simulink model "DT"  (R2025b)
settings: Solver=ode5  StartTime=0.0  StopTime=inf  RelTol=1e-3
InitFcn:
  | PLC_IP = "10.10.6.1";
  | port_num = 502;
  | 
  | 
  | load("macierze_do_modelu.mat")
undefined symbols (not defined in the file or in its folder): dol_p1, dol_p2, dol_p3, flows_diff, gora_p1, gora_p2, gora_p3, lvls, M_cofka, M_pump_A1, online, pompa_sterowanie, pump_a1_delay_a, pump_a1_delay_b, pump_a2_delay_a, pump_a2_delay_b, R1_K_dol, R1_K_gora, R1_sterowanie, R2_K_dol, R2_K_gora, R2_od_dolu, R2_od_gory, R2_sterowanie, R3, R4, R5, R6, R7, rozgalezienie_h1_dol, rozgalezienie_h1_gora, rozgalezienie_h2_dol, rozgalezienie_h2_gora, rozgalezienie_korekta_A1_dol, rozgalezienie_korekta_A2_dol, sterowanie, V_max, V_out_max
libraries: modbuslib x5, simulink x2, sldrtlib x1
settings Model: ParamWorkspaceSource=ReferencedWorkspace  TunableVars=R4,R3,R5,R6,R7,R8,R1_sterowanie,R2_sterowanie,pompa_sterowanie  TunableVarsStorageClass=Auto,Auto,Auto,Auto,Auto,Auto,Auto,Auto,Auto  TunableVarsTypeQualifier=,,,,,,,,  Creator=Ania  LastModifiedBy=student
settings DebuggingCC: UnderspecifiedInitializationDetection=Classic  MergeDetectMultiDrivingBlocksExec=none
settings HardwareCC: ProdBitPerLong=64.0  ProdHWDeviceType=Intel->x86-64 (Linux 64)
settings ModelReferenceCC: PropagateSignalLabelsOutOfModel=off
settings RTWCC: SystemTargetFile=sldrt.tlc  TemplateMakefile=sldrt.tmf  RTWCompilerOptimization=on  Description=Simulink Desktop Real-Time
settings CodeAppCC: MaxIdLength=95.0
settings SimulinkDesktopRealTimeCC: ExtModeTransport=0.0  ExtModeStaticAllocSize=1000000.0  TargetLibSuffix=_sldrt.a  TargetPreCompLibLocation=C:\Program Files\MATLAB\R2025b\toolbox\sldrt\lib\win64  MultiwordLength=2048.0  DynamicStringBufferSize=256.0  ParMdlRefBuildCompliant=on  PreserveMATLABNamespacesInGeneratedCode=on  SubcomponentCodeInterfacePackaging=Reusable function

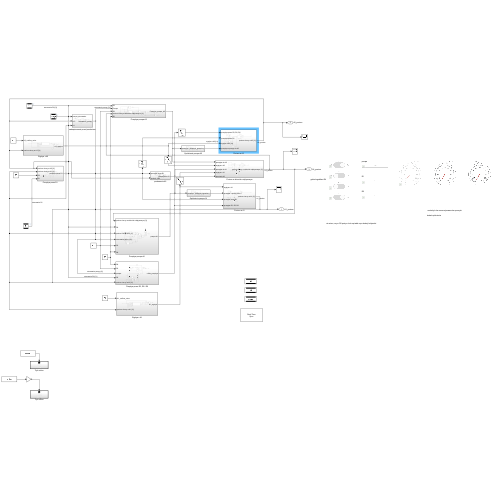
[thumbnail: Simulink's stored preview of the top-level diagram]
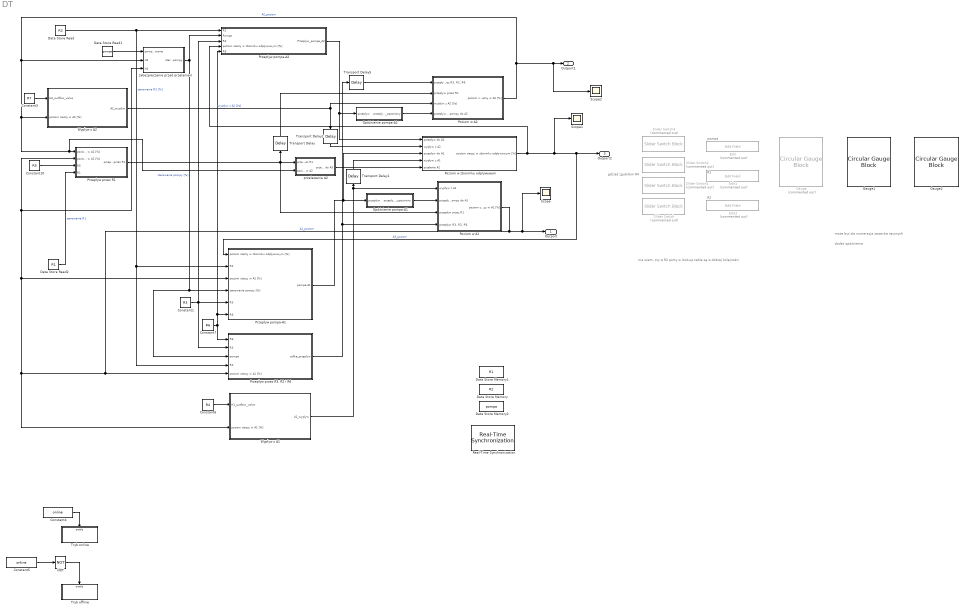
== system DT ==
  note: nie wiem, czy w R2 porty w look-up table są w dobrej kolejności
  note: dodać opóźnienia
  note: gdzieś zgubiłam R4
  note: R2
  note: R1
  note: pompa
  note: może być zła numeracja zaworów ręcznych
  Constant1 : Constant  Value=R3  OutDataTypeStr=boolean
  Constant10 : Constant  Value=R5  OutDataTypeStr=boolean
  Constant3 : Constant  Value=R7  OutDataTypeStr=boolean
  Constant4 : Constant  Value=online  OutDataTypeStr=boolean
  Constant5 : Constant  Value=online  OutDataTypeStr=boolean
  Constant6 : Constant  Value=R4  OutDataTypeStr=boolean
  Constant7 : Constant  Value=R6  OutDataTypeStr=boolean
  Data Store Memory : DataStoreMemory  DataStoreName=R2  WriteAfterWriteMsg=warning  ShowAdditionalParam=off
  Data Store Memory1 : DataStoreMemory  DataStoreName=R1  WriteAfterWriteMsg=warning  ShowAdditionalParam=off
  Data Store Memory2 : DataStoreMemory  DataStoreName=pompa  WriteAfterWriteMsg=warning  ShowAdditionalParam=off
  Data Store Read : DataStoreRead  DataStoreName=R2  IndexOptions=Index vector (dialog)  Indices=1  OutputSizes=1
  Data Store Read1 : DataStoreRead  DataStoreName=pompa  IndexOptions=Index vector (dialog)  Indices=1  OutputSizes=1
  Data Store Read2 : DataStoreRead  DataStoreName=R1  IndexOptions=Index vector (dialog)  Indices=1  OutputSizes=1
  Edit : EditField  Commented=on  LabelPosition=Hide  ShowInitialText=on  Alignment=Center
  Edit1 : EditField  Commented=on  LabelPosition=Hide  ShowInitialText=on  Alignment=Center
  Edit2 : EditField  Commented=on  LabelPosition=Hide  ShowInitialText=on  Alignment=Center
  Gauge : CircularGaugeBlock  Commented=on  FontColor=[0.0, 0.0, 0.0]
  Gauge1 : CircularGaugeBlock  FontColor=[0.0, 0.0, 0.0]
  Gauge2 : CircularGaugeBlock  FontColor=[0.0, 0.0, 0.0]
  NOT : Logic  Operator=NOT  IconShape=distinctive  AllPortsSameDT=off  OutDataTypeStr=boolean
  Opóźnienie pompa-A1 : Subsystem
  Opóźnienie pompa-A2 : Subsystem
  Poziom w A1 : Subsystem
  Poziom w A2 : Subsystem
  Poziom w zbiorniku odplywowym : Subsystem
  Przepływ pompa-A1 : Subsystem
  Przepływ pompa-A2 : Subsystem
  Przepływ przez R1 : Subsystem
  "Przepływ przez R3, R2 i R6" : Subsystem
  Real-Time Synchronization : sldrtlib/Real-Time Synchronization  SampleTime=0.1  MaxMissedTicks=5000  ShowMissedTicks=off  YieldWhenWaiting=off
  Scope : Scope
      settings: DataLoggingSaveFormat=Array
  Scope1 : Scope
      settings: DataLoggingSaveFormat=Array
  Scope2 : Scope
      settings: DataLoggingVariableName=ScopeData2  DataLoggingSaveFormat=Array
  Slider Switch{,1..2,4} (4 alike) : SliderSwitchBlock  Commented=on
  Transport Delay : TransportDelay  DelayTime=1.65
  Transport Delay1 : TransportDelay  DelayTime=1.15
  Transport Delay2 : TransportDelay  DelayTime=0.9
  Transport Delay5 : TransportDelay  DelayTime=2
  Tryb offline : Subsystem  TreatAsAtomicUnit=on
  Tryb online : Subsystem  TreatAsAtomicUnit=on
  Wypływ z A1 : Subsystem
  Wypływ z A2 : Subsystem
  przelewanie A2 : Subsystem
  zabezpieczenie przed przelaniem : Subsystem
  Outport : Outport  SignalName=A1_poziom
  Outport1 : Outport  Port=2  SignalName=A2_poziom
  Outport2 : Outport  Port=3  SignalName=A3_poziom
  wires:
  Data Store Read/1 -> "Przepływ przez R3, R2 i R6"/4(R2), Przepływ pompa-A1/2(R2), Przepływ pompa-A2/1(R2)  "sterowanie R2 [%]"
  Przepływ pompa-A2/1(Przeplyw_pompa_A2) -> Poziom w zbiorniku odplywowym/1(przepływ do A2), Opóźnienie pompa-A2/1(przeplyw)
  Wypływ z A2/1(A2_wypływ) -> Poziom w A2/3(wypływ z A2 [l/s]), Transport Delay2/1  "wypływ z A2 [l/s]"
  Constant3/1 -> Wypływ z A2/1(H2_outflow_valve)
  Wypływ z A1/1(A1_wyplyw) -> Poziom w A1/1(wypływ z A1), Transport Delay1/1
  Constant6/1 -> Wypływ z A1/1(H1_outflow_valve)
  "Przepływ przez R3, R2 i R6"/1(cofka_przeplyw) -> Transport Delay5/1, Poziom w A1/4("przepływ R3, R2, R6")
  Constant7/1 -> "Przepływ przez R3, R2 i R6"/1(R6), Przepływ pompa-A2/5(R6), Przepływ pompa-A1/6(R6)
  Przepływ pompa-A1/1(pompa-A1) -> Poziom w zbiorniku odplywowym/3(przepływ do A1), Opóźnienie pompa-A1/1(przeplyw)
  Data Store Read2/1 -> Przepływ przez R1/4(R1)  "sterowanie R1"
  Przepływ przez R1/1(przepływ przez R1) -> Transport Delay/1, Poziom w A1/3(przepływ przez R1), przelewanie A2/1(przepływ przez R1)
  Constant10/1 -> Przepływ przez R1/3(R5)
  Poziom w A1/1(poziom cieczy w A1 [%]) -> "Przepływ przez R3, R2 i R6"/5(poziom cieczy w A1 [%]), Przepływ przez R1/2(poziom cieczy w A1 [%]), zabezpieczenie przed przelaniem/3(H1), Przepływ pompa-A1/3(poziom cieczy w A1 [%]), Wypływ z A1/2(poziom cieczy w A1 [%]), Scope/1, Outport/1  "A1_poziom"
  Poziom w A2/1(poziom cieczy w A2 [%]) -> Scope2/1, Outport1/1, Wypływ z A2/2(poziom cieczy w A2 [%]), Przepływ przez R1/1(poziom cieczy w A2 [%]), przelewanie A2/2(poziom w A2), zabezpieczenie przed przelaniem/2(H2)  "A2_poziom"
  Poziom w zbiorniku odplywowym/1(poziom cieczy w zbiorniku odpływowym [%]) -> Scope1/1, Przepływ pompa-A1/1(poziom cieczy w zbiorniku odpływowym [%]), Outport2/1, Przepływ pompa-A2/4(poziom cieczy w zbiorniku odpływowym [%])  "A3_poziom"
  Constant1/1 -> "Przepływ przez R3, R2 i R6"/2(R3), Przepływ pompa-A2/3(R3), Przepływ pompa-A1/5(R3)
  zabezpieczenie przed przelaniem/1(sterowanie_pompy) -> "Przepływ przez R3, R2 i R6"/3(pompa), Przepływ pompa-A1/4(sterowanie pompy [%]), Przepływ pompa-A2/2(Pompa)  "sterowanie pompy [%]"
  Data Store Read1/1 -> zabezpieczenie przed przelaniem/1(pompa_sterowanie)
  przelewanie A2/1(przepływ do A3) -> Poziom w zbiorniku odplywowym/5(przelanie A2)
  Transport Delay/1 -> Poziom w A2/2(przepływ przez R1)
  Transport Delay1/1 -> Poziom w zbiorniku odplywowym/4(wypływ z A1)
  Transport Delay2/1 -> Poziom w zbiorniku odplywowym/2(wypływ z A2)
  Opóźnienie pompa-A2/1(przeplyw_opozniony) -> Poziom w A2/4(przepływ z pompy do A2)
  Opóźnienie pompa-A1/1(przeplyw_opozniony) -> Poziom w A1/2(przepływ z pompy do A1)
  Transport Delay5/1 -> Poziom w A2/1("przepływ przez R3, R2, R6")
  Constant4/1 -> Tryb online/Enable
  NOT/1 -> Tryb offline/Enable
  Constant5/1 -> NOT/1

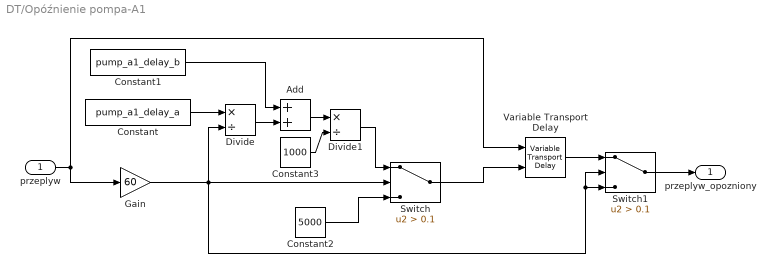
== system DT/Opóźnienie pompa-A1 ==
  przeplyw : Inport
  Add : Sum
  Constant : Constant  Value=pump_a1_delay_a
  Constant1 : Constant  Value=pump_a1_delay_b
  Constant2 : Constant  Value=5000
  Constant3 : Constant  Value=1000
  Divide : Product  Inputs=*/
  Divide1 : Product  Inputs=*/
  Gain : Gain  Gain=60
  Switch : Switch  Criteria=u2 > Threshold  Threshold=0.1  SaturateOnIntegerOverflow=off  InputSameDT=off
  Switch1 : Switch  Criteria=u2 > Threshold  Threshold=0.1  SaturateOnIntegerOverflow=off  InputSameDT=off
  Variable Transport Delay : VariableTransportDelay  VariableDelayType=Variable transport delay  MaximumDelay=5000
  przeplyw_opozniony : Outport
  wires:
  Constant/1 -> Divide/1
  przeplyw/1 -> Gain/1, Variable Transport Delay/1
  Divide/1 -> Add/2
  Constant1/1 -> Add/1
  Constant2/1 -> Switch/3
  Switch/1 -> Variable Transport Delay/2
  Add/1 -> Divide1/1
  Divide1/1 -> Switch/1
  Constant3/1 -> Divide1/2
  Gain/1 -> Switch/2, Switch1/3, Switch1/2, Divide/2
  Variable Transport Delay/1 -> Switch1/1
  Switch1/1 -> przeplyw_opozniony/1

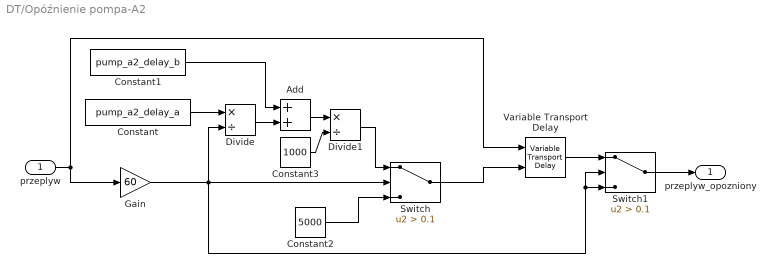
== system DT/Opóźnienie pompa-A2 ==
  przeplyw : Inport
  Add : Sum
  Constant : Constant  Value=pump_a2_delay_a
  Constant1 : Constant  Value=pump_a2_delay_b
  Constant2 : Constant  Value=5000
  Constant3 : Constant  Value=1000
  Divide : Product  Inputs=*/
  Divide1 : Product  Inputs=*/
  Gain : Gain  Gain=60
  Switch : Switch  Criteria=u2 > Threshold  Threshold=0.1  SaturateOnIntegerOverflow=off  InputSameDT=off
  Switch1 : Switch  Criteria=u2 > Threshold  Threshold=0.1  SaturateOnIntegerOverflow=off  InputSameDT=off
  Variable Transport Delay : VariableTransportDelay  VariableDelayType=Variable transport delay  MaximumDelay=5000
  przeplyw_opozniony : Outport
  wires:
  Switch1/1 -> przeplyw_opozniony/1
  Variable Transport Delay/1 -> Switch1/1
  Gain/1 -> Divide/2, Switch1/2, Switch1/3, Switch/2
  Constant3/1 -> Divide1/2
  Divide1/1 -> Switch/1
  Add/1 -> Divide1/1
  Switch/1 -> Variable Transport Delay/2
  Constant2/1 -> Switch/3
  Constant1/1 -> Add/1
  Divide/1 -> Add/2
  przeplyw/1 -> Variable Transport Delay/1, Gain/1
  Constant/1 -> Divide/1

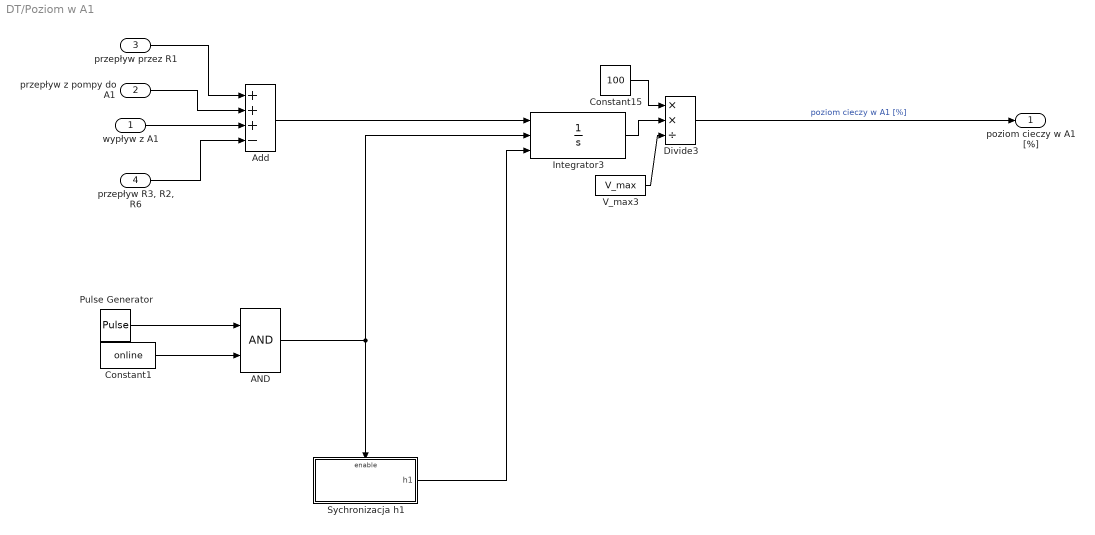
== system DT/Poziom w A1 ==
  wypływ z A1 : Inport
  przepływ z pompy do A1 : Inport  Port=2
  przepływ przez R1 : Inport  Port=3
  "przepływ R3, R2, R6" : Inport  Port=4
  AND : Logic  IconShape=distinctive  AllPortsSameDT=off  OutDataTypeStr=boolean
  Add : Sum  Inputs=+++-
  Constant1 : Constant  Value=online  OutDataTypeStr=boolean
  Constant15 : Constant  Value=100
  Divide3 : Product  Inputs=**/
  Integrator3 : Integrator  ExternalReset=rising  InitialConditionSource=external  LimitOutput=on  UpperSaturationLimit=V_max  LowerSaturationLimit=0
  Pulse Generator : DiscretePulseGenerator  PulseType=Time based  Period=60  PulseWidth=5
  Sychronizacja h1 : Subsystem  TreatAsAtomicUnit=on
  V_max3 : Constant  Value=V_max
  poziom cieczy w A1 [%] : Outport
  wires:
  wypływ z A1/1 -> Add/3
  przepływ z pompy do A1/1 -> Add/2
  Add/1 -> Integrator3/1
  Integrator3/1 -> Divide3/2
  Constant15/1 -> Divide3/1
  Divide3/1 -> poziom cieczy w A1 [%]/1  "poziom cieczy w A1 [%]"
  V_max3/1 -> Divide3/3
  "przepływ R3, R2, R6"/1 -> Add/4
  przepływ przez R1/1 -> Add/1
  Sychronizacja h1/1(h1) -> Integrator3/3
  Constant1/1 -> AND/2
  AND/1 -> Integrator3/2, Sychronizacja h1/Enable
  Pulse Generator/1 -> AND/1

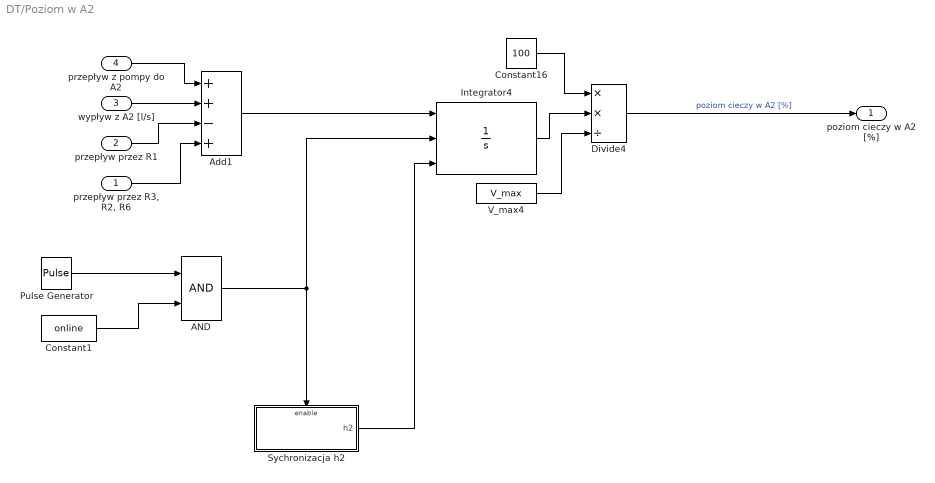
== system DT/Poziom w A2 ==
  "przepływ przez R3, R2, R6" : Inport
  przepływ przez R1 : Inport  Port=2
  wypływ z A2 [l/s] : Inport  Port=3
  przepływ z pompy do A2 : Inport  Port=4
  AND : Logic  IconShape=distinctive  AllPortsSameDT=off  OutDataTypeStr=boolean
  Add1 : Sum  Inputs=++-+
  Constant1 : Constant  Value=online  OutDataTypeStr=boolean
  Constant16 : Constant  Value=100
  Divide4 : Product  Inputs=**/
  Integrator4 : Integrator  ExternalReset=rising  InitialConditionSource=external  LimitOutput=on  UpperSaturationLimit=V_max  LowerSaturationLimit=0
  Pulse Generator : DiscretePulseGenerator  PulseType=Time based  Period=60  PulseWidth=5
  Sychronizacja h2 : Subsystem  TreatAsAtomicUnit=on
  V_max4 : Constant  Value=V_max
  poziom cieczy w A2 [%] : Outport
  wires:
  "przepływ przez R3, R2, R6"/1 -> Add1/4
  V_max4/1 -> Divide4/3
  Integrator4/1 -> Divide4/2
  wypływ z A2 [l/s]/1 -> Add1/2
  Divide4/1 -> poziom cieczy w A2 [%]/1  "poziom cieczy w A2 [%]"
  Add1/1 -> Integrator4/1
  Constant16/1 -> Divide4/1
  przepływ z pompy do A2/1 -> Add1/1
  przepływ przez R1/1 -> Add1/3
  Pulse Generator/1 -> AND/1
  Constant1/1 -> AND/2
  AND/1 -> Integrator4/2, Sychronizacja h2/Enable
  Sychronizacja h2/1(h2) -> Integrator4/3

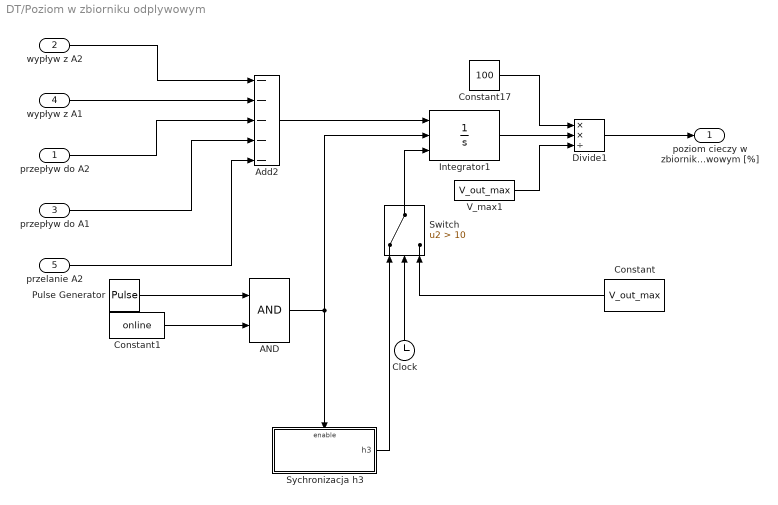
== system DT/Poziom w zbiorniku odplywowym ==
  przepływ do A2 : Inport
  wypływ z A2 : Inport  Port=2
  przepływ do A1 : Inport  Port=3
  wypływ z A1 : Inport  Port=4
  przelanie A2 : Inport  Port=5
  AND : Logic  IconShape=distinctive  AllPortsSameDT=off  OutDataTypeStr=boolean
  Add2 : Sum  Inputs=-----
  Clock : Clock
  Constant : Constant  Value=V_out_max
  Constant1 : Constant  Value=online  OutDataTypeStr=boolean
  Constant17 : Constant  Value=100
  Divide1 : Product  Inputs=**/
  Integrator1 : Integrator  ExternalReset=rising  InitialConditionSource=external  InitialCondition=V_out_max  LimitOutput=on  UpperSaturationLimit=V_out_max  LowerSaturationLimit=0
  Pulse Generator : DiscretePulseGenerator  PulseType=Time based  Period=60  PulseWidth=5
  Switch : Switch  Criteria=u2 > Threshold  Threshold=10  SaturateOnIntegerOverflow=off  InputSameDT=off
  Sychronizacja h3 : Subsystem  TreatAsAtomicUnit=on
  V_max1 : Constant  Value=V_out_max  OutDataTypeStr=double
  poziom cieczy w zbiorniku odpływowym [%] : Outport
  wires:
  Add2/1 -> Integrator1/1
  V_max1/1 -> Divide1/3
  Integrator1/1 -> Divide1/2
  przepływ do A1/1 -> Add2/4
  Constant17/1 -> Divide1/1
  wypływ z A1/1 -> Add2/2
  Divide1/1 -> poziom cieczy w zbiorniku odpływowym [%]/1
  przepływ do A2/1 -> Add2/3
  wypływ z A2/1 -> Add2/1
  przelanie A2/1 -> Add2/5
  Constant1/1 -> AND/2
  AND/1 -> Sychronizacja h3/Enable, Integrator1/2
  Pulse Generator/1 -> AND/1
  Sychronizacja h3/1(h3) -> Switch/1
  Switch/1 -> Integrator1/3
  Constant/1 -> Switch/3
  Clock/1 -> Switch/2

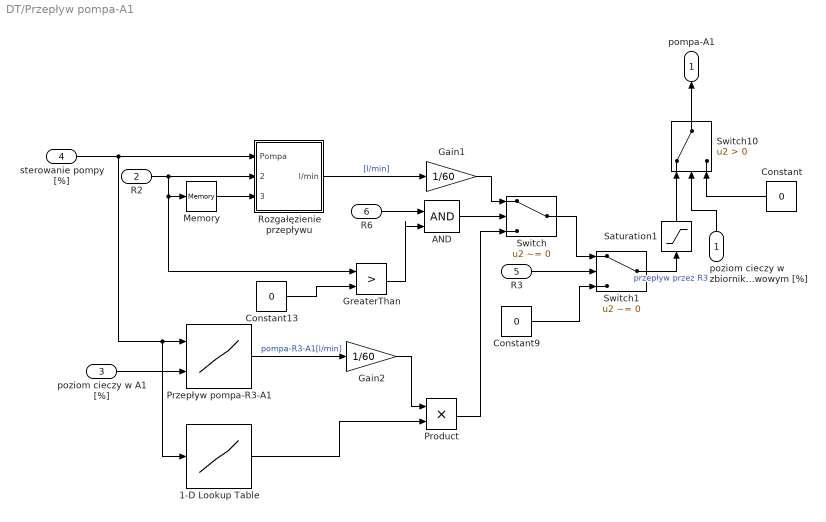
== system DT/Przepływ pompa-A1 ==
  poziom cieczy w zbiorniku odpływowym [%] : Inport
  R2 : Inport  Port=2
  poziom cieczy w A1 [%] : Inport  Port=3
  sterowanie pompy [%] : Inport  Port=4
  R3 : Inport  Port=5
  R6 : Inport  Port=6
  1-D Lookup Table : Lookup_n-D  NumberOfTableDimensions=1  BreakpointsForDimension1=[30, 40, 60, 80, 100]  Table=[1, 1.0243, 1.0582, 1.0915, 1.0664]  InternalRulePriority=Speed  RndMeth=Simplest
  AND : Logic  IconShape=distinctive  AllPortsSameDT=off  OutDataTypeStr=boolean
  Constant : Constant  Value=0
  Constant13 : Constant  Value=0  OutDataTypeStr=double
  Constant9 : Constant  Value=0  OutDataTypeStr=double
  Gain1 : Gain  Gain=1/60
  Gain2 : Gain  Gain=1/60
  GreaterThan : RelationalOperator  Operator=>  OutDataTypeStr=boolean  RndMeth=Simplest  InputSameDT=off
  Memory : Memory
  Product : Product
  Przepływ pompa-R3-A1 : Lookup_n-D  BreakpointsForDimension1=40:10:100  BreakpointsForDimension2=0:10:100  IndexSearchMethod=Linear search  Table=M_pump_A1'  InternalRulePriority=Speed  RndMeth=Simplest
      settings: InputPortMap=u0,u1
  Rozgałęzienie przepływu : Subsystem
  Saturation1 : Saturate  UpperLimit=35  LowerLimit=0
  Switch : Switch  Criteria=u2 ~= 0  SaturateOnIntegerOverflow=off  InputSameDT=off
  Switch1 : Switch  Criteria=u2 ~= 0  SaturateOnIntegerOverflow=off  InputSameDT=off
  Switch10 : Switch  Criteria=u2 > Threshold  SaturateOnIntegerOverflow=off  InputSameDT=off
  pompa-A1 : Outport
  wires:
  R6/1 -> AND/1
  Switch1/1 -> Saturation1/1  "przepływ przez R3"
  R2/1 -> Rozgałęzienie przepływu/2(Zawor2), Memory/1, GreaterThan/1
  Constant9/1 -> Switch1/3
  Switch10/1 -> pompa-A1/1
  R3/1 -> Switch1/2
  Memory/1 -> Rozgałęzienie przepływu/3(Zawor2_prev)
  Constant/1 -> Switch10/3
  AND/1 -> Switch/2
  poziom cieczy w A1 [%]/1 -> Przepływ pompa-R3-A1/2
  Rozgałęzienie przepływu/1(l/min) -> Gain1/1  "[l/min]"
  sterowanie pompy [%]/1 -> Rozgałęzienie przepływu/1(Pompa), 1-D Lookup Table/1, Przepływ pompa-R3-A1/1
  1-D Lookup Table/1 -> Product/2
  Switch/1 -> Switch1/1
  Gain1/1 -> Switch/1
  Przepływ pompa-R3-A1/1 -> Gain2/1  "pompa-R3-A1[l/min]"
  Saturation1/1 -> Switch10/1
  GreaterThan/1 -> AND/2
  poziom cieczy w zbiorniku odpływowym [%]/1 -> Switch10/2
  Gain2/1 -> Product/1
  Constant13/1 -> GreaterThan/2
  Product/1 -> Switch/3

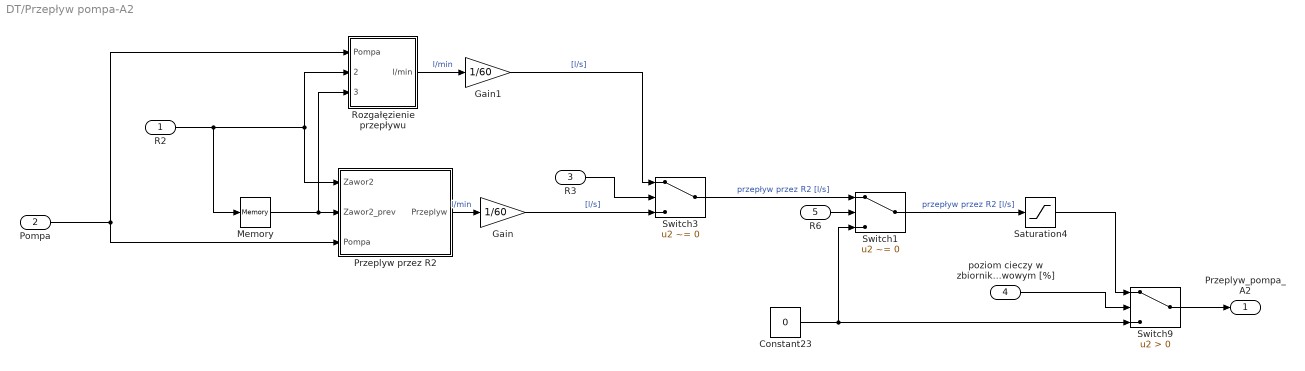
== system DT/Przepływ pompa-A2 ==
  R2 : Inport
  Pompa : Inport  Port=2
  R3 : Inport  Port=3
  poziom cieczy w zbiorniku odpływowym [%] : Inport  Port=4
  R6 : Inport  Port=5
  Constant23 : Constant  Value=0
  Gain : Gain  Gain=1/60
  Gain1 : Gain  Gain=1/60
  Memory : Memory
  Przeplyw przez R2 : Subsystem
  Rozgałęzienie przepływu : Subsystem
  Saturation4 : Saturate  UpperLimit=35  LowerLimit=0
  Switch1 : Switch  Criteria=u2 ~= 0  SaturateOnIntegerOverflow=off  InputSameDT=off
  Switch3 : Switch  Criteria=u2 ~= 0  SaturateOnIntegerOverflow=off  InputSameDT=off
  Switch9 : Switch  Criteria=u2 > Threshold  SaturateOnIntegerOverflow=off  InputSameDT=off
  Przeplyw_pompa_A2 : Outport
  wires:
  Pompa/1 -> Rozgałęzienie przepływu/1(Pompa), Przeplyw przez R2/3(Pompa)
  Saturation4/1 -> Switch9/1
  Przeplyw przez R2/1(Przeplyw) -> Gain/1  "l/min"
  Gain1/1 -> Switch3/1  "[l/s]"
  Gain/1 -> Switch3/3  "[l/s]"
  Rozgałęzienie przepływu/1(l/min) -> Gain1/1  "l/min"
  Constant23/1 -> Switch9/3, Switch1/3
  R2/1 -> Memory/1, Rozgałęzienie przepływu/2(Zawor2), Przeplyw przez R2/1(Zawor2)
  Switch9/1 -> Przeplyw_pompa_A2/1
  poziom cieczy w zbiorniku odpływowym [%]/1 -> Switch9/2
  R3/1 -> Switch3/2
  R6/1 -> Switch1/2
  Switch3/1 -> Switch1/1  "przepływ przez R2 [l/s]"
  Switch1/1 -> Saturation4/1  "przepływ przez R2 [l/s]"
  Memory/1 -> Rozgałęzienie przepływu/3(Zawor2_prev), Przeplyw przez R2/2(Zawor2_prev)

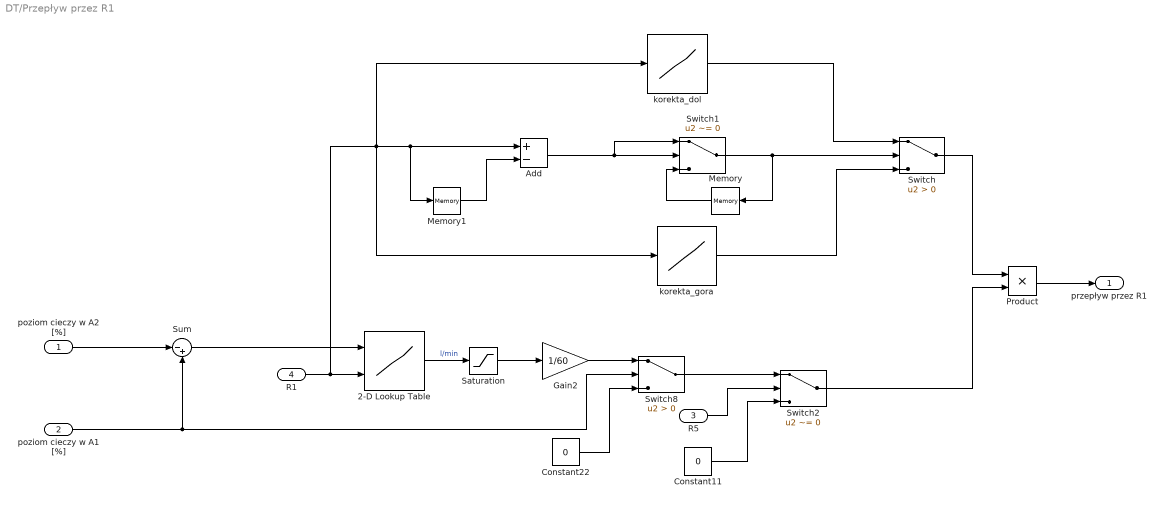
== system DT/Przepływ przez R1 ==
  poziom cieczy w A2 [%] : Inport
  poziom cieczy w A1 [%] : Inport  Port=2
  R5 : Inport  Port=3
  R1 : Inport  Port=4
  2-D Lookup Table : Lookup_n-D  BreakpointsForDimension1=lvls  BreakpointsForDimension2=40:10:100  Table=flows_diff  InterpMethod=Cubic spline  ExtrapMethod=Cubic spline  InternalRulePriority=Speed  RndMeth=Simplest
      settings: InputPortMap=u0,u1
  Add : Sum  Inputs=+-
  Constant11 : Constant  Value=0  OutDataTypeStr=double
  Constant22 : Constant  Value=0
  Gain2 : Gain  Gain=1/60
  Memory : Memory
  Memory1 : Memory
  Product : Product
  Saturation : Saturate  UpperLimit=0  LowerLimit=-35
  Sum : Sum  Inputs=|-+
  Switch : Switch  Criteria=u2 > Threshold  SaturateOnIntegerOverflow=off  InputSameDT=off
  Switch1 : Switch  Criteria=u2 ~= 0  SaturateOnIntegerOverflow=off  InputSameDT=off
  Switch2 : Switch  Criteria=u2 ~= 0  SaturateOnIntegerOverflow=off  InputSameDT=off
  Switch8 : Switch  Criteria=u2 > Threshold  SaturateOnIntegerOverflow=off  InputSameDT=off
  korekta_dol : Lookup_n-D  NumberOfTableDimensions=1  BreakpointsForDimension1=40:10:100  Table=R1_K_dol  InternalRulePriority=Speed  RndMeth=Simplest
  korekta_gora : Lookup_n-D  NumberOfTableDimensions=1  BreakpointsForDimension1=40:10:100  Table=R1_K_gora  InternalRulePriority=Speed  RndMeth=Simplest
  przepływ przez R1 : Outport
  wires:
  2-D Lookup Table/1 -> Saturation/1  "l/min"
  Sum/1 -> 2-D Lookup Table/1
  korekta_dol/1 -> Switch/1
  R5/1 -> Switch2/2
  Gain2/1 -> Switch8/1
  poziom cieczy w A1 [%]/1 -> Sum/2, Switch8/2
  Memory1/1 -> Add/2
  korekta_gora/1 -> Switch/3
  Memory/1 -> Switch1/3
  Product/1 -> przepływ przez R1/1
  Constant11/1 -> Switch2/3
  R1/1 -> korekta_gora/1, korekta_dol/1, Memory1/1, Add/1, 2-D Lookup Table/2
  poziom cieczy w A2 [%]/1 -> Sum/1
  Switch/1 -> Product/1
  Saturation/1 -> Gain2/1
  Switch2/1 -> Product/2
  Switch8/1 -> Switch2/1
  Constant22/1 -> Switch8/3
  Switch1/1 -> Switch/2, Memory/1
  Add/1 -> Switch1/1, Switch1/2

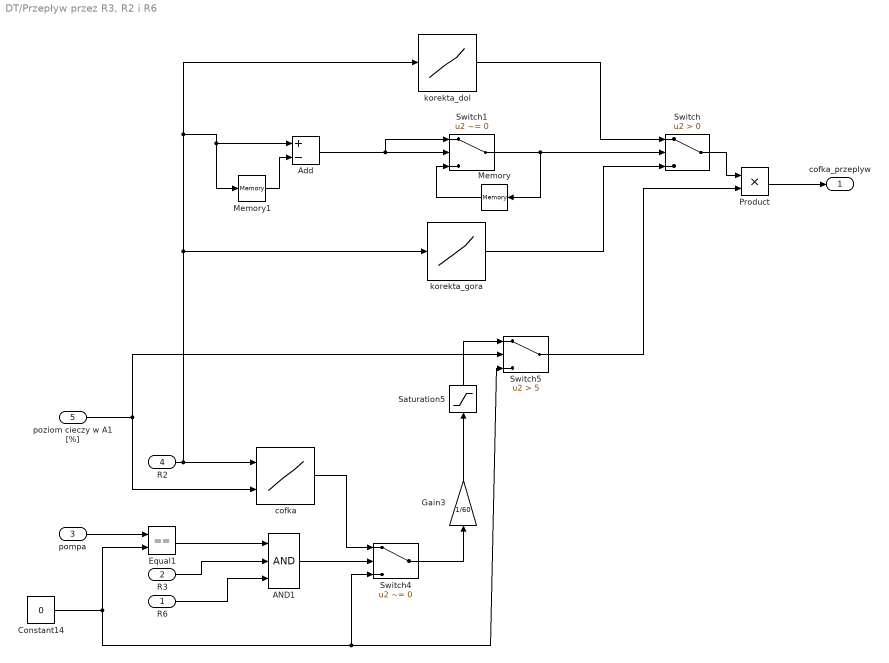
== system DT/Przepływ przez R3, R2 i R6 ==
  R6 : Inport
  R3 : Inport  Port=2
  pompa : Inport  Port=3
  R2 : Inport  Port=4
  poziom cieczy w A1 [%] : Inport  Port=5
  AND1 : Logic  Inputs=3  IconShape=distinctive  AllPortsSameDT=off  OutDataTypeStr=boolean
  Add : Sum  Inputs=+-
  Constant14 : Constant  Value=0
  Equal1 : RelationalOperator  Operator===  OutDataTypeStr=boolean  RndMeth=Simplest  InputSameDT=off
  Gain3 : Gain  Gain=1/60
  Memory : Memory
  Memory1 : Memory
  Product : Product
  Saturation5 : Saturate  UpperLimit=35  LowerLimit=0
  Switch : Switch  Criteria=u2 > Threshold  SaturateOnIntegerOverflow=off  InputSameDT=off
  Switch1 : Switch  Criteria=u2 ~= 0  SaturateOnIntegerOverflow=off  InputSameDT=off
  Switch4 : Switch  Criteria=u2 ~= 0  SaturateOnIntegerOverflow=off  InputSameDT=off
  Switch5 : Switch  Criteria=u2 > Threshold  Threshold=5  SaturateOnIntegerOverflow=off  InputSameDT=off
  cofka : Lookup_n-D  BreakpointsForDimension1=30:10:100  BreakpointsForDimension2=10:10:100  Table=M_cofka  InternalRulePriority=Speed  RndMeth=Simplest
      settings: InputPortMap=u0,u1
  korekta_dol : Lookup_n-D  NumberOfTableDimensions=1  BreakpointsForDimension1=40:10:100  Table=[0.56, 1, 1, 1, 1, 1, 1]  InternalRulePriority=Speed  RndMeth=Simplest
  korekta_gora : Lookup_n-D  NumberOfTableDimensions=1  BreakpointsForDimension1=40:10:100  Table=[1, 1.18, 1, 1, 1, 1, 1]  InternalRulePriority=Speed  RndMeth=Simplest
  cofka_przeplyw : Outport
  wires:
  R6/1 -> AND1/3
  Switch1/1 -> Switch/2, Memory/1
  Switch5/1 -> Product/2
  Switch/1 -> Product/1
  korekta_gora/1 -> Switch/3
  Add/1 -> Switch1/1, Switch1/2
  Memory/1 -> Switch1/3
  AND1/1 -> Switch4/2
  R3/1 -> AND1/2
  Switch4/1 -> Gain3/1
  korekta_dol/1 -> Switch/1
  Product/1 -> cofka_przeplyw/1
  Constant14/1 -> Equal1/2, Switch4/3, Switch5/3
  Equal1/1 -> AND1/1
  Saturation5/1 -> Switch5/1
  pompa/1 -> Equal1/1
  poziom cieczy w A1 [%]/1 -> Switch5/2, cofka/2
  R2/1 -> cofka/1, korekta_dol/1, Memory1/1, Add/1, korekta_gora/1
  Memory1/1 -> Add/2
  cofka/1 -> Switch4/1
  Gain3/1 -> Saturation5/1

== system DT/Tryb offline ==
  Enable : EnablePort
  Constant : Constant  Value=pompa_sterowanie  OutDataTypeStr=double
  Constant2 : Constant  Value=R1_sterowanie
  Data Store Write : DataStoreWrite  DataStoreName=R2  IndexOptions=Index vector (dialog)  Indices=1  OutputSizes=1
  Data Store Write1 : DataStoreWrite  DataStoreName=R1  IndexOptions=Index vector (dialog)  Indices=1  OutputSizes=1
  Data Store Write2 : DataStoreWrite  DataStoreName=pompa  IndexOptions=Index vector (dialog)  Indices=1  OutputSizes=1
  Wartosc zadana R2 : Constant  Value=R2_sterowanie  OutMin=0  OutMax=100
  wires:
  Wartosc zadana R2/1 -> Data Store Write/1  "sterowanie R2 [%]"
  Constant/1 -> Data Store Write2/1
  Constant2/1 -> Data Store Write1/1

== system DT/Tryb online ==
  Enable : EnablePort
  Constant4 : Constant  Value=sterowanie  OutDataTypeStr=boolean
  Constant5 : Constant  Value=sterowanie  OutDataTypeStr=boolean
  NOT : Logic  Operator=NOT  IconShape=distinctive  AllPortsSameDT=off  OutDataTypeStr=boolean
  Tryb monitorowania : Subsystem  TreatAsAtomicUnit=on
  Tryb sterowania : Subsystem  TreatAsAtomicUnit=on
  wires:
  NOT/1 -> Tryb monitorowania/Enable
  Constant4/1 -> Tryb sterowania/Enable
  Constant5/1 -> NOT/1

== system DT/Wypływ z A1 ==
  H1_outflow_valve : Inport
  poziom cieczy w A1 [%] : Inport  Port=2
  Constant : Constant  Value=gora_p1
  Constant1 : Constant  Value=gora_p2
  Constant2 : Constant  Value=gora_p3
  Constant20 : Constant  Value=0  OutDataTypeStr=double
  Constant3 : Constant  Value=V_max
  Saturation2 : Saturate  UpperLimit=0  LowerLimit=-35
  Switch6 : Switch  Criteria=u2 > Threshold  SaturateOnIntegerOverflow=off  InputSameDT=off
  Wypływ z A1 : MATLAB Function  TreatAsAtomicUnit=on
  A1_wyplyw : Outport
  wires:
  Switch6/1 -> A1_wyplyw/1
  Wypływ z A1/1(flow) -> Saturation2/1  "wypływ góra [l/s]"
  Constant20/1 -> Switch6/3
  Saturation2/1 -> Switch6/1
  H1_outflow_valve/1 -> Wypływ z A1/1(H1_outflow_valve)
  poziom cieczy w A1 [%]/1 -> Switch6/2, Wypływ z A1/2(H1_lvl)
  Constant/1 -> Wypływ z A1/3(p1)
  Constant1/1 -> Wypływ z A1/4(p2)
  Constant2/1 -> Wypływ z A1/5(p3)
  Constant3/1 -> Wypływ z A1/6(V_max)

== system DT/Wypływ z A2 ==
  H2_outflow_valve : Inport
  poziom cieczy w A2 [%] : Inport  Port=2
  Constant : Constant  Value=dol_p1
  Constant1 : Constant  Value=dol_p2
  Constant2 : Constant  Value=dol_p3
  Constant21 : Constant  Value=0
  Constant3 : Constant  Value=V_max
  Saturation3 : Saturate  UpperLimit=0  LowerLimit=-35
  Switch7 : Switch  Criteria=u2 > Threshold  SaturateOnIntegerOverflow=off  InputSameDT=off
  Wypływ z A2 : MATLAB Function  TreatAsAtomicUnit=on
  A2_wypływ : Outport
  wires:
  Wypływ z A2/1(flow) -> Saturation3/1  "wypływ dół [l/s]"
  Saturation3/1 -> Switch7/1
  H2_outflow_valve/1 -> Wypływ z A2/1(H2_outflow_valve)
  poziom cieczy w A2 [%]/1 -> Switch7/2, Wypływ z A2/2(H2_lvl)
  Switch7/1 -> A2_wypływ/1
  Constant21/1 -> Switch7/3
  Constant/1 -> Wypływ z A2/3(p1)
  Constant3/1 -> Wypływ z A2/6(V_max)
  Constant2/1 -> Wypływ z A2/5(p3)
  Constant1/1 -> Wypływ z A2/4(p2)

== system DT/przelewanie A2 ==
  przepływ przez R1 : Inport
  poziom w A2 : Inport  Port=2
  Constant4 : Constant  Value=0
  Switch : Switch  Threshold=100  SaturateOnIntegerOverflow=off  InputSameDT=off
  przepływ do A3 : Outport
  wires:
  Switch/1 -> przepływ do A3/1
  przepływ przez R1/1 -> Switch/1
  Constant4/1 -> Switch/3
  poziom w A2/1 -> Switch/2

== system DT/zabezpieczenie przed przelaniem ==
  pompa_sterowanie : Inport
  H2 : Inport  Port=2
  H1 : Inport  Port=3
  AND : Logic  IconShape=distinctive  AllPortsSameDT=off  OutDataTypeStr=boolean
  Compare To Constant : simulink/Logic and Bit Operations/Compare To Constant  relop=<  const=100  OutDataTypeStr=boolean
  Compare To Constant1 : simulink/Logic and Bit Operations/Compare To Constant  relop=<  const=100  OutDataTypeStr=boolean
  Constant4 : Constant  Value=0
  Scope : Scope
      settings: DataLoggingSaveFormat=Array
  Switch : Switch  Criteria=u2 ~= 0  Threshold=100  SaturateOnIntegerOverflow=off  InputSameDT=off
  sterowanie_pompy : Outport
  wires:
  H1/1 -> Compare To Constant/1
  Constant4/1 -> Switch/3
  Compare To Constant1/1 -> AND/2
  AND/1 -> Scope/1, Switch/2  "zabezpieczenie_warunek"
  Compare To Constant/1 -> AND/1
  H2/1 -> Compare To Constant1/1
  pompa_sterowanie/1 -> Switch/1
  Switch/1 -> sterowanie_pompy/1

== system DT/Poziom w A1/Sychronizacja h1 ==
  Enable : EnablePort
  Gain : Gain  Gain=V_max/100
  Modbus Client Read : modbuslib/Modbus Client Read  RetainClient=PLC  ClientList=PLC  ConnectionEndpoint=10.10.6.1:2000  ServerId=1  RegisterTable={ '1', 'h1', '7', 'Holding Register', 'uint16', '1' }  SampleTime=-1
  h1 : Outport
  wires:
  Modbus Client Read/1 -> Gain/1
  Gain/1 -> h1/1

== system DT/Poziom w A2/Sychronizacja h2 ==
  Enable : EnablePort
  Gain : Gain  Gain=V_max/100
  Modbus Client Read : modbuslib/Modbus Client Read  RetainClient=PLC  ClientList=PLC  ConnectionEndpoint=10.10.6.1:2000  ServerId=1  RegisterTable={ '1', 'h2', '9', 'Holding Register', 'uint16', '1' }  SampleTime=-1
  h2 : Outport
  wires:
  Modbus Client Read/1 -> Gain/1
  Gain/1 -> h2/1

== system DT/Poziom w zbiorniku odplywowym/Sychronizacja h3 ==
  Enable : EnablePort
  Constant : Constant  Value=V_out_max
  Gain : Gain  Gain=V_max/100
  Gain1 : Gain  Gain=V_max/100
  Minus : Sum  Inputs=+--
  Modbus Client Read : modbuslib/Modbus Client Read  RetainClient=PLC  ClientList=PLC  ConnectionEndpoint=10.10.6.1:2000  ServerId=1  RegisterTable={ '1', 'h1', '7', 'Holding Register', 'uint16', '1'; '2', 'h2', '9', 'Holding Register', 'uint16', '1' }  SampleTime=-1
  h3 : Outport
  wires:
  Modbus Client Read/1 -> Gain/1
  Modbus Client Read/2 -> Gain1/1
  Gain/1 -> Minus/2
  Gain1/1 -> Minus/3
  Minus/1 -> h3/1
  Constant/1 -> Minus/1

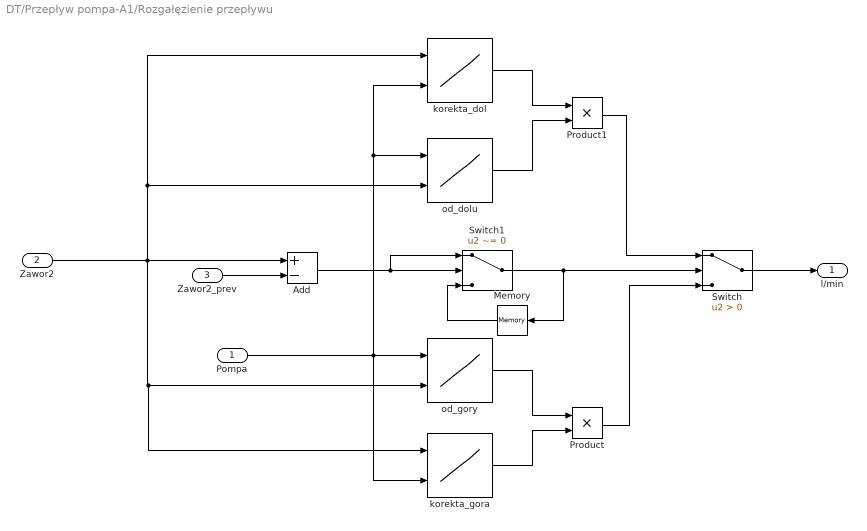
== system DT/Przepływ pompa-A1/Rozgałęzienie przepływu ==
  Pompa : Inport
  Zawor2 : Inport  Port=2
  Zawor2_prev : Inport  Port=3
  Add : Sum  Inputs=+-
  Memory : Memory
  Product : Product
  Product1 : Product
  Switch : Switch  Criteria=u2 > Threshold  SaturateOnIntegerOverflow=off  InputSameDT=off
  Switch1 : Switch  Criteria=u2 ~= 0  SaturateOnIntegerOverflow=off  InputSameDT=off
  korekta_dol : Lookup_n-D  BreakpointsForDimension1=30:10:100  BreakpointsForDimension2=40:10:100  Table=rozgalezienie_korekta_A1_dol  InternalRulePriority=Speed  RndMeth=Simplest
      settings: InputPortMap=u0,u1
  korekta_gora : Lookup_n-D  BreakpointsForDimension1=30:10:100  BreakpointsForDimension2=40:10:100  Table=rozgalezienie_korekta_A2_dol  InternalRulePriority=Speed  RndMeth=Simplest
      settings: InputPortMap=u0,u1
  od_dolu : Lookup_n-D  BreakpointsForDimension1=40:10:100  BreakpointsForDimension2=30:10:100  Table=rozgalezienie_h1_dol  InternalRulePriority=Speed  RndMeth=Simplest
      settings: InputPortMap=u0,u1
  od_gory : Lookup_n-D  BreakpointsForDimension1=40:10:100  BreakpointsForDimension2=30:10:100  Table=rozgalezienie_h1_gora  InternalRulePriority=Speed  RndMeth=Simplest
      settings: InputPortMap=u0,u1
  l/min : Outport
  wires:
  Add/1 -> Switch1/1, Switch1/2
  Product1/1 -> Switch/1
  Product/1 -> Switch/3
  Switch1/1 -> Switch/2, Memory/1
  Switch/1 -> l/min/1
  Zawor2_prev/1 -> Add/2
  Zawor2/1 -> korekta_gora/1, od_gory/2, korekta_dol/1, od_dolu/2, Add/1
  Pompa/1 -> korekta_gora/2, od_gory/1, korekta_dol/2, od_dolu/1
  Memory/1 -> Switch1/3
  korekta_dol/1 -> Product1/1
  od_dolu/1 -> Product1/2
  od_gory/1 -> Product/1
  korekta_gora/1 -> Product/2

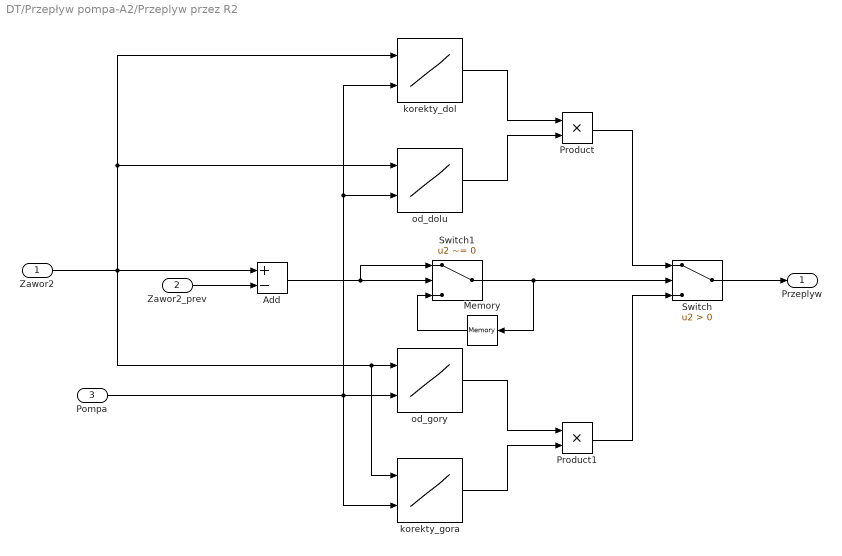
== system DT/Przepływ pompa-A2/Przeplyw przez R2 ==
  Zawor2 : Inport
  Zawor2_prev : Inport  Port=2
  Pompa : Inport  Port=3
  Add : Sum  Inputs=+-
  Memory : Memory
  Product : Product
  Product1 : Product
  Switch : Switch  Criteria=u2 > Threshold  SaturateOnIntegerOverflow=off  InputSameDT=off
  Switch1 : Switch  Criteria=u2 ~= 0  SaturateOnIntegerOverflow=off  InputSameDT=off
  korekty_dol : Lookup_n-D  BreakpointsForDimension1=0:10:100  BreakpointsForDimension2=0:10:100  Table=R2_K_dol  InternalRulePriority=Speed  RndMeth=Simplest
      settings: InputPortMap=u0,u1
  korekty_gora : Lookup_n-D  BreakpointsForDimension1=0:10:100  BreakpointsForDimension2=0:10:100  Table=R2_K_gora  InternalRulePriority=Speed  RndMeth=Simplest
      settings: InputPortMap=u0,u1
  od_dolu : Lookup_n-D  BreakpointsForDimension1=0:10:100  BreakpointsForDimension2=0:10:100  Table=R2_od_dolu  InternalRulePriority=Speed  RndMeth=Simplest
      settings: InputPortMap=u0,u1
  od_gory : Lookup_n-D  BreakpointsForDimension1=0:10:100  BreakpointsForDimension2=0:10:100  Table=R2_od_gory  InternalRulePriority=Speed  RndMeth=Simplest
      settings: InputPortMap=u0,u1
  Przeplyw : Outport
  wires:
  Switch1/1 -> Switch/2, Memory/1
  Add/1 -> Switch1/1, Switch1/2
  Product/1 -> Switch/1
  Zawor2/1 -> korekty_gora/1, od_gory/1, Add/1, od_dolu/1, korekty_dol/1
  od_dolu/1 -> Product/2
  korekty_gora/1 -> Product1/2
  Switch/1 -> Przeplyw/1
  Zawor2_prev/1 -> Add/2
  Pompa/1 -> korekty_gora/2, od_gory/2, korekty_dol/2, od_dolu/2
  Memory/1 -> Switch1/3
  od_gory/1 -> Product1/1
  korekty_dol/1 -> Product/1
  Product1/1 -> Switch/3

== system DT/Przepływ pompa-A2/Rozgałęzienie przepływu ==
  Pompa : Inport
  Zawor2 : Inport  Port=2
  Zawor2_prev : Inport  Port=3
  Add : Sum  Inputs=+-
  Memory : Memory
  Switch : Switch  Criteria=u2 > Threshold  SaturateOnIntegerOverflow=off  InputSameDT=off
  Switch1 : Switch  Criteria=u2 ~= 0  SaturateOnIntegerOverflow=off  InputSameDT=off
  od_dolu : Lookup_n-D  BreakpointsForDimension1=40:10:100  BreakpointsForDimension2=30:10:100  Table=rozgalezienie_h2_dol  InternalRulePriority=Speed  RndMeth=Simplest
      settings: InputPortMap=u0,u1
  od_gory : Lookup_n-D  BreakpointsForDimension1=40:10:100  BreakpointsForDimension2=30:10:100  Table=rozgalezienie_h2_gora  InternalRulePriority=Speed  RndMeth=Simplest
      settings: InputPortMap=u0,u1
  l/min : Outport
  wires:
  Add/1 -> Switch1/1, Switch1/2
  od_dolu/1 -> Switch/1
  od_gory/1 -> Switch/3
  Switch1/1 -> Switch/2, Memory/1
  Switch/1 -> l/min/1
  Zawor2_prev/1 -> Add/2
  Zawor2/1 -> od_gory/2, od_dolu/2, Add/1
  Pompa/1 -> od_gory/1, od_dolu/1
  Memory/1 -> Switch1/3

== system DT/Tryb online/Tryb monitorowania ==
  Enable : EnablePort
  Data Store Write : DataStoreWrite  DataStoreName=pompa  IndexOptions=Index vector (dialog)  Indices=1  OutputSizes=1
  Data Store Write1 : DataStoreWrite  DataStoreName=R1  IndexOptions=Index vector (dialog)  Indices=1  OutputSizes=1
  Data Store Write2 : DataStoreWrite  DataStoreName=R2  IndexOptions=Index vector (dialog)  Indices=1  OutputSizes=1
  Gain : Gain  Gain=1/100
  Gain1 : Gain  Gain=1/100
  Gain2 : Gain  Gain=1/100
  Modbus Client Read : modbuslib/Modbus Client Read  RetainClient=PLC  ClientList=PLC  ConnectionEndpoint=10.10.6.1:2000  ServerId=1  RegisterTable={ '1', 'pompa', '1207', 'Holding Register', 'uint16', '1'; '2', 'R1', '1201', 'Holding Register', 'uint16', '1'; '3', 'R2', '1203', 'Holding Register', 'uint16', '1' }  SampleTime=-1
  wires:
  Modbus Client Read/1 -> Gain/1
  Modbus Client Read/2 -> Gain1/1
  Modbus Client Read/3 -> Gain2/1
  Gain/1 -> Data Store Write/1
  Gain1/1 -> Data Store Write1/1
  Gain2/1 -> Data Store Write2/1

== system DT/Tryb online/Tryb sterowania ==
  Enable : EnablePort
  Constant : Constant  Value=pompa_sterowanie  OutDataTypeStr=double
  Constant2 : Constant  Value=R1_sterowanie
  Constant3 : Constant  Value=R2_sterowanie  OutMin=0  OutMax=100
  Data Store Write : DataStoreWrite  DataStoreName=R2  IndexOptions=Index vector (dialog)  Indices=1  OutputSizes=1
  Data Store Write1 : DataStoreWrite  DataStoreName=R1  IndexOptions=Index vector (dialog)  Indices=1  OutputSizes=1
  Data Store Write2 : DataStoreWrite  DataStoreName=pompa  IndexOptions=Index vector (dialog)  Indices=1  OutputSizes=1
  Gain : Gain  Gain=100
  Gain1 : Gain  Gain=100
  Gain2 : Gain  Gain=100
  Modbus Client Write : modbuslib/Modbus Client Write  RetainClient=PLC  ClientList=PLC  ConnectionEndpoint=10.10.6.1:2000  ServerId=1  RegisterTable={ '1', 'pompa', '1207', 'Holding Register', 'uint16'; '2', 'R1', '1201', 'Holding Register', 'uint16'; '3', 'R2', '1203', 'Holding Register', 'uint16' }  SampleTime=-1
  wires:
  Constant2/1 -> Gain1/1, Data Store Write1/1
  Constant/1 -> Gain/1, Data Store Write2/1
  Constant3/1 -> Data Store Write/1, Gain2/1
  Gain/1 -> Modbus Client Write/1
  Gain1/1 -> Modbus Client Write/2
  Gain2/1 -> Modbus Client Write/3

== matlab function DT/Wypływ z A2/Wypływ z A2 ==
  data: H2_outflow_valve input; flow output; H2_lvl input; p1 input; p2 input; p3 input; V_max input
function flow = H2_outflow(H2_outflow_valve, H2_lvl, p1, p2, p3, V_max)
    flow = 0.0;
    if H2_outflow_valve == 1
        t = (-p2-sqrt(p2^2-4*p1*(p3-H2_lvl)))/(2*p1);

        dol_odplyw_value = 2*p1*t + p2;
        
        % Użycie tej wartości w finalnym obliczeniu:
        flow = V_max * dol_odplyw_value / 100; 
    else
        flow = 0;
    end
end

== matlab function DT/Wypływ z A1/Wypływ z A1 ==
  data: H1_outflow_valve input; flow output; H1_lvl input; p1 input double; p2 input double; p3 input double; V_max input
function flow = H1_outflow(H1_outflow_valve, H1_lvl, p1, p2, p3, V_max)
flow = 0.0;
    if H1_outflow_valve == 1
        t = (-p2-sqrt(p2^2-4*p1*(p3-H1_lvl)))/(2*p1);
        
        gora_odplyw_value = 2*p1*t + p2;
        
        flow = V_max * gora_odplyw_value / 100; 
    else
        flow = 0.0;
    end
end
